simulink model "Lab1_before_PID"  (R2014b)
settings: Solver=ode45  StartTime=0.0  StopTime=10.0  RelTol=1e-3
undefined symbols (not defined in the file): b, g, I, l, M, m
settings Model: Creator=nrjbasu  LastModifiedBy=nrjbasu
settings DebuggingCC: AlgebraicLoopMsg=none

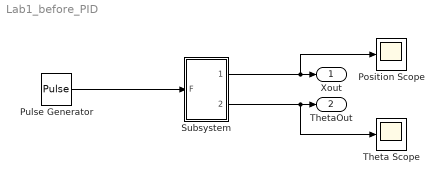
== system Lab1_before_PID ==
  Position Scope : Scope
      settings: TimeRange=10  YMin=0  YMax=60000
  Pulse Generator : DiscretePulseGenerator  PulseType=Time based  Amplitude=1000  Period=10  PulseWidth=.001
  Subsystem : Subsystem
  Theta Scope : Scope
  Xout : Outport
  ThetaOut : Outport  Port=2
  wires:
  Subsystem/2(Out2) -> Theta Scope/1, ThetaOut/1
  Subsystem/1(Out1) -> Position Scope/1, Xout/1
  Pulse Generator/1 -> Subsystem/1(F)

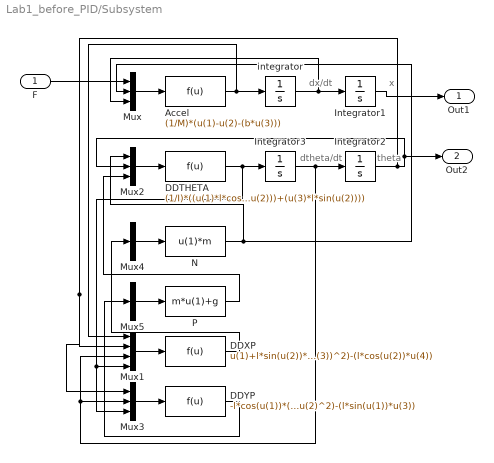
== system Lab1_before_PID/Subsystem ==
  note: x
  note: theta
  note: dtheta/dt
  note: dx/dt
  F : Inport
  Accel : Fcn  Expr=(1/M)*(u(1)-u(2)-(b*u(3)))
  DDTHETA : Fcn  Expr=(1/I)*((u(1)*l*cos(u(2)))+(u(3)*l*sin(u(2))))
  DDXP : Fcn  Expr=u(1)+l*sin(u(2))*((u(3))^2)-(l*cos(u(2))*u(4))
  DDYP : Fcn  Expr=-l*cos(u(1))*(u(2)^2)-(l*sin(u(1))*u(3))
  Integrator1 : Integrator
  Integrator2 : Integrator  InitialCondition=pi
  Integrator3 : Integrator
  Mux : Mux  Inputs=3
  Mux1 : Mux
  Mux2 : Mux  Inputs=3
  Mux3 : Mux  Inputs=3
  Mux4 : Mux  Inputs=1
  Mux5 : Mux  Inputs=1
  N : Fcn  Expr=u(1)*m
  P : Fcn  Expr=m*u(1)+g
  integrator : Integrator
  Out1 : Outport
  Out2 : Outport  Port=2
  wires:
  P/1 -> Mux2/3
  F/1 -> Mux/1
  N/1 -> Mux2/1, Mux/2
  Integrator1/1 -> Out1/1
  DDTHETA/1 -> Mux1/4, Mux3/3, Integrator3/1
  Accel/1 -> Mux1/1, integrator/1
  Integrator2/1 -> Mux3/1, Mux1/2, Out2/1, Mux2/2
  Integrator3/1 -> Mux3/2, Mux1/3, Integrator2/1
  Mux/1 -> Accel/1
  Mux3/1 -> DDYP/1
  Mux2/1 -> DDTHETA/1
  Mux1/1 -> DDXP/1
  integrator/1 -> Mux/3, Integrator1/1
  Mux4/1 -> N/1
  Mux5/1 -> P/1
  DDXP/1 -> Mux4/1
  DDYP/1 -> Mux5/1
